simulink model "impulse"  (R2022b)
settings: Solver=VariableStepAuto  StartTime=0.0  StopTime=10.0  RelTol=1e-3
settings Model: Creator=wojna  LastModifiedBy=wojna

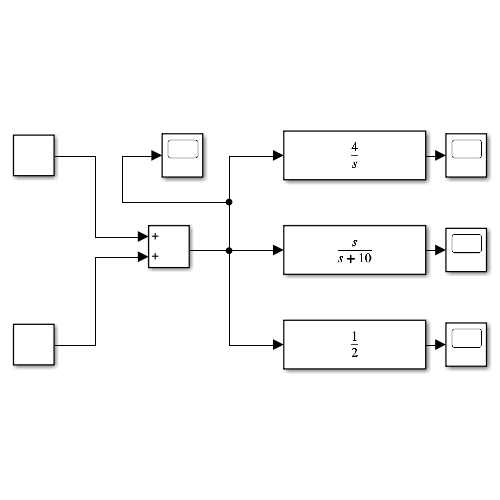
[thumbnail: Simulink's stored preview of the top-level diagram]
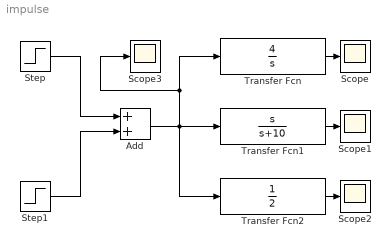
== system impulse ==
  Add : Sum
  Scope{,1..3} (4 alike) : Scope
  Step : Step  SampleTime=0
  Step1 : Step  Time=1.01  After=-1  SampleTime=0
  Transfer Fcn : TransferFcn  Numerator=[4]  Denominator=[1 0]
  Transfer Fcn1 : TransferFcn  Numerator=[1 0]  Denominator=[1 10]
  Transfer Fcn2 : TransferFcn  Denominator=[0 2]
  wires:
  Step/1 -> Add/1
  Step1/1 -> Add/2
  Add/1 -> Scope3/1, Transfer Fcn/1, Transfer Fcn2/1, Transfer Fcn1/1
  Transfer Fcn/1 -> Scope/1
  Transfer Fcn1/1 -> Scope1/1
  Transfer Fcn2/1 -> Scope2/1
